simulink model "demostration"  (R2014b)
settings: Solver=ode45  StartTime=0.0  StopTime=10  RelTol=1e-3
settings Model: Creator=wangze  LastModifiedBy=jonesdm
settings OptimizationCC: UseDivisionForNetSlopeComputation=off  SimCompilerOptimization=off
settings DebuggingCC: FrameProcessingCompatibilityMsg=error  AllowSymbolicDim=off
settings RTWCC: RTWCompilerOptimization=off
settings ConfigComp: CovMetricSettings=dw  CovHtmlReporting=on  CovSaveCumulativeToWorkspaceVar=on  CovSaveSingleToWorkspaceVar=on  CovModelRefEnable=Off  CovExternalEMLEnable=off  CovSFcnEnable=off

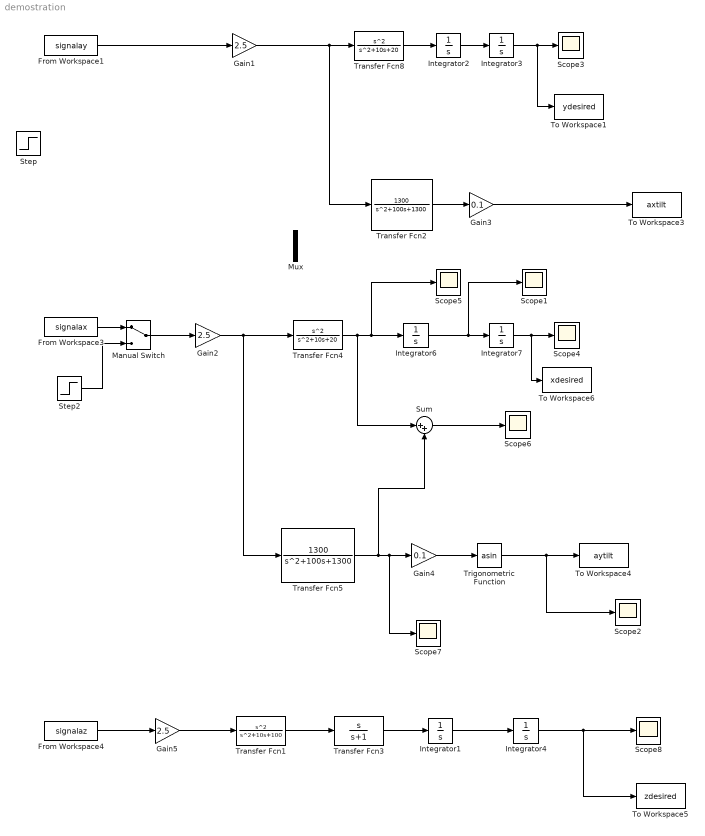
== system demostration ==
  From Workspace1 : FromWorkspace  VariableName=signalay  SampleTime=0
  From Workspace3 : FromWorkspace  VariableName=signalax  SampleTime=0.05
  From Workspace4 : FromWorkspace  VariableName=signalaz  SampleTime=0.05
  Gain1 : Gain  Gain=2.5  SampleTime=0.05
  Gain2 : Gain  Gain=2.5  SampleTime=0.05
  Gain3 : Gain  Gain=0.1  SampleTime=0.05
  Gain4 : Gain  Gain=0.1  SampleTime=0.05
  Gain5 : Gain  Gain=2.5  SampleTime=0.05
  Integrator{1..4,6..7} (6 alike) : Integrator
  Manual Switch : ManualSwitch
  Mux : Mux  Inputs=2
  Scope{1..8} (8 alike) : Scope
      Scope1 settings: YMin=-0.28187  YMax=0.50005
      Scope2 settings: YMin=-0.61859  YMax=5.56733
      Scope4 settings: YMin=-0.02793  YMax=0.23064  SaveName=ScopeData4
      Scope5 settings: YMin=-4.15952  YMax=4.62545  SaveName=ScopeData5
      Scope6 settings: YMin=-1.35826  YMax=8.01741  SaveName=ScopeData6
      Scope7 settings: YMin=-1.04879  YMax=7.28512  SaveName=ScopeData7
  Step : Step  SampleTime=0
  Step2 : Step  Time=0  SampleTime=0
  Sum : Sum  Inputs=|++
  To Workspace1 : ToWorkspace  VariableName=ydesired  SampleTime=0.05
      settings: Decimation=2  Save2DSignal=2-D array (concatenate along first dimension)
  To Workspace3 : ToWorkspace  VariableName=axtilt  SampleTime=-1
      settings: Decimation=2
  To Workspace4 : ToWorkspace  VariableName=aytilt  SampleTime=-1
      settings: Decimation=2
  To Workspace5 : ToWorkspace  VariableName=zdesired  SampleTime=-1
      settings: Decimation=2
  To Workspace6 : ToWorkspace  VariableName=xdesired  SampleTime=0.05
      settings: Decimation=2  Save2DSignal=2-D array (concatenate along first dimension)
  Transfer Fcn1 : TransferFcn  Numerator=[1 0 0]  Denominator=[1 10 100]
  Transfer Fcn2 : TransferFcn  Numerator=[1300]  Denominator=[1 100 1300]
  Transfer Fcn3 : TransferFcn  Numerator=[1 0]  Denominator=[1 1]
  Transfer Fcn4 : TransferFcn  Numerator=[1 0 0]  Denominator=[1 10 20]
  Transfer Fcn5 : TransferFcn  Numerator=[1300]  Denominator=[1 100 1300]
  Transfer Fcn8 : TransferFcn  Numerator=[1 0 0]  Denominator=[1 10 20]
  Trigonometric Function : Trigonometry  Operator=asin
  wires:
  Integrator2/1 -> Integrator3/1
  Integrator3/1 -> Scope3/1, To Workspace1/1
  Integrator6/1 -> Scope1/1, Integrator7/1
  Transfer Fcn4/1 -> Sum/1, Scope5/1, Integrator6/1
  Integrator7/1 -> To Workspace6/1, Scope4/1
  Gain1/1 -> Transfer Fcn2/1, Transfer Fcn8/1
  Gain4/1 -> Trigonometric Function/1
  Transfer Fcn5/1 -> Sum/2, Scope7/1, Gain4/1
  Gain2/1 -> Transfer Fcn5/1, Transfer Fcn4/1
  Manual Switch/1 -> Gain2/1
  From Workspace1/1 -> Gain1/1
  Transfer Fcn8/1 -> Integrator2/1
  From Workspace4/1 -> Gain5/1
  Gain5/1 -> Transfer Fcn1/1
  Transfer Fcn1/1 -> Transfer Fcn3/1
  Transfer Fcn3/1 -> Integrator1/1
  Integrator1/1 -> Integrator4/1
  Integrator4/1 -> To Workspace5/1, Scope8/1
  Step2/1 -> Manual Switch/2
  From Workspace3/1 -> Manual Switch/1
  Sum/1 -> Scope6/1
  Transfer Fcn2/1 -> Gain3/1
  Gain3/1 -> To Workspace3/1
  Trigonometric Function/1 -> Scope2/1, To Workspace4/1
